simulink model "labeca_simulink_2021a"  (R2021a)
settings: Solver=VariableStepAuto  StartTime=0.0  StopTime=0.6  RelTol=1e-3
values from neighbouring files (symbols this model uses):
  ganho_K = step_resposta/step_excitacao    [labeca.m]    (also in resposta_ao_degrau.m)
  tau_area = A0/(media_canal2_sup - media_canal2_inf)    [labeca.m]    (also in resposta_ao_degrau.m)
  tau_nep = 1 / a    [labeca.m]    (also in resposta_ao_degrau.m)
settings Model: Creator=helenabrener  LastModifiedBy=caioc
settings DebuggingCC: UnconnectedInputMsg=none  UnconnectedOutputMsg=none  UnconnectedLineMsg=none
settings ModelReferenceCC: EnableRefExpFcnMdlSchedulingChecks=off
settings RTWCC: Description=Generic Real-Time Target  DLArmComputeVersion=20.02.1

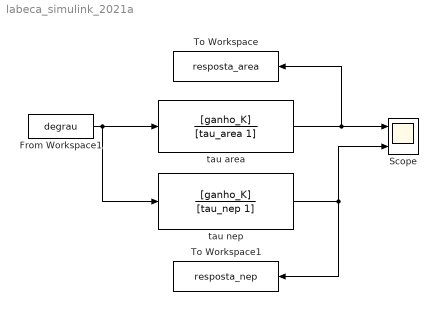
== system labeca_simulink_2021a ==
  " tau area" : TransferFcn  Numerator=[ganho_K]  Denominator=[tau_area 1]
  From Workspace1 : FromWorkspace  VariableName=degrau
  Scope : Scope  NumInputPorts=2
  To Workspace : ToWorkspace  VariableName=resposta_area  SaveFormat=Timeseries  SampleTime=-1
  To Workspace1 : ToWorkspace  VariableName=resposta_nep  SaveFormat=Timeseries  SampleTime=-1
  tau nep : TransferFcn  Numerator=[ganho_K]  Denominator=[tau_nep 1]
  wires:
  " tau area"/1 -> Scope/1, To Workspace/1
  tau nep/1 -> Scope/2, To Workspace1/1
  From Workspace1/1 -> tau nep/1, " tau area"/1
